simulink model "HW7_v2"  (R2019b)
settings: Solver=VariableStepAuto  StartTime=0.0  StopTime=15  RelTol=1e-3
values from neighbouring files (symbols this model uses):
  A1_wiener = [0 1 ;               0 0]    [HW7_v2_matlab.m]
  A2_cont = [0]    [HW7_v2_matlab.m]
  B1_wiener = [0;               1]    [HW7_v2_matlab.m]
  B2_cont = [1]    [HW7_v2_matlab.m]
  C1_wiener = [1 0]    [HW7_v2_matlab.m]
  C2_cont = [1]    [HW7_v2_matlab.m]
  D1_wiener = [0]    [HW7_v2_matlab.m]
  D2_cont = [0]    [HW7_v2_matlab.m]
  L1 = lqe(A1_cont, G1, C1_cont, Q1, R1, N1)    [HW7_v2_matlab.m]
  L2 = lqe(A2_cont, G2, C2_cont, Q2, R2, N2)    [HW7_v2_matlab.m]
  L3 = lqe(A2_cont, G2, C2_cont, Q3, R3, N3)    [HW7_v2_matlab.m]
  L4 = lqe(A2_cont, G2, C2_cont, Q4, R4, N4)    [HW7_v2_matlab.m]
  L5 = lqe(A2_cont, G2, C2_cont, Q5, R5, N5)    [HW7_v2_matlab.m]
  M_inv = inv(M_motor)    [HW7_v2_matlab.m]
  M_motor = [1, 1, 1, -1;             1, 1, -1, 1;             1, -1, -1, -1;             1, -1, 1, 1 ]    [HW7_v2_matlab.m]
  measurement_noise = 0.1    [kalman_matrices_calculator.m]
  tau2 = eval(max(solve(1/sqrt((tau2*2*pi*10)^2+1^2) == 1/sqrt(2), tau2)))    [HW7_v2_matlab.m]    (also in kalman_matrices_calculator.m = 0.0159154943092)
  V = 5    [HW7_v2_matlab.m]
  V0 = 5    [HW7_v2_matlab.m]
undefined symbols (not defined in the file or in its folder): A, A1, A3, A4, Aaileron, Aelevator, Arudder, Athrust, B, B1, B3, B4, Baileron, Belevator, Brudder, Bthrust, C, C1, C3, C4, Caileron, Celevator, Crudder, Cthrust, D, D1, D3, D4, Daileron, Delevator, DiscIntNeverNeededParam, Drudder, Dthrust, K2, K3, K4, Kx1, trim_state
libraries: simulink x1
(part 2 of 2)

== system HW7_v2/Nonlinear System/vdot ==
  theta : Inport
  phi : Inport  Port=2
  p : Inport  Port=3
  w : Inport  Port=4
  r : Inport  Port=5
  u : Inport  Port=6
  Constant : Constant  Value=9.81  SampleTime=0.05
  Cos : Trigonometry  Operator=cos
  Integrator5 : Integrator
  Product : Product  Inputs=3
  Sin : Trigonometry
  Sum : Sum  Inputs=+-+
  p*w : Product
  r*u : Product
  v : Outport
  wires:
  r/1 -> r*u/1
  p/1 -> p*w/1
  Sum/1 -> Integrator5/1
  Integrator5/1 -> v/1  "v"
  w/1 -> p*w/2
  u/1 -> r*u/2
  r*u/1 -> Sum/3
  theta/1 -> Cos/1
  Cos/1 -> Product/2
  Sin/1 -> Product/3
  phi/1 -> Sin/1
  Product/1 -> Sum/1
  p*w/1 -> Sum/2
  Constant/1 -> Product/1

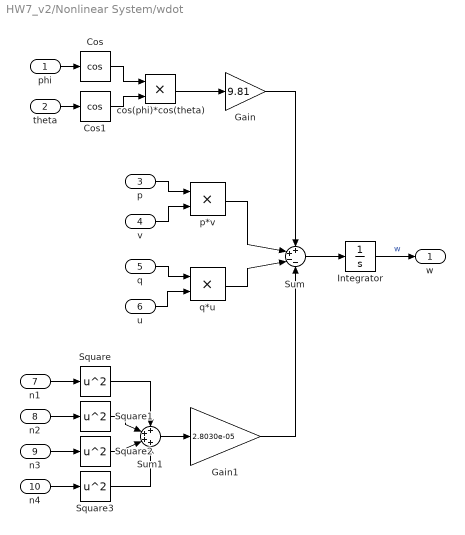
== system HW7_v2/Nonlinear System/wdot  ==
  phi : Inport
  theta : Inport  Port=2
  p : Inport  Port=3
  v : Inport  Port=4
  q : Inport  Port=5
  u : Inport  Port=6
  n1 : Inport  Port=7
  n2 : Inport  Port=8
  n3 : Inport  Port=9
  n4 : Inport  Port=10
  Cos : Trigonometry  Operator=cos
  Cos1 : Trigonometry  Operator=cos
  Gain : Gain  Gain=9.81
  Gain1 : Gain  Gain=2.8030e-05
  Integrator : Integrator
  Square{,1..3} (4 alike) : Math  Operator=square  SignedPower=off  SaturateOnIntegerOverflow=on
  Sum : Sum  Inputs=++--
  Sum1 : Sum  Inputs=++++
  cos(phi)*cos(theta) : Product
  p*v : Product
  q*u : Product
  w : Outport
  wires:
  q*u/1 -> Sum/3
  u/1 -> q*u/2
  Integrator/1 -> w/1  "w"
  Gain/1 -> Sum/1
  q/1 -> q*u/1
  Sum/1 -> Integrator/1
  v/1 -> p*v/2
  p/1 -> p*v/1
  p*v/1 -> Sum/2
  theta/1 -> Cos1/1
  Cos1/1 -> cos(phi)*cos(theta)/2
  Cos/1 -> cos(phi)*cos(theta)/1
  cos(phi)*cos(theta)/1 -> Gain/1
  phi/1 -> Cos/1
  n1/1 -> Square/1
  Gain1/1 -> Sum/4
  Square/1 -> Sum1/1
  n2/1 -> Square1/1
  n3/1 -> Square2/1
  n4/1 -> Square3/1
  Square1/1 -> Sum1/2
  Square2/1 -> Sum1/3
  Square3/1 -> Sum1/4
  Sum1/1 -> Gain1/1
